simulink model "Ambient_TestBed_org"  (Simulink 10.0)
settings: Solver=FixedStepDiscrete  StartTime=0.0  StopTime=1  FixedStep=1  RelTol=1e-3  EnableMultiTasking=on
undefined symbols (not defined in the file): MWS
libraries: Lib_Turbo_Ambient_TMATS x1
settings Model: Creator=jwchapm2  LastModifiedBy=bhisma
settings DataIOCC: LimitDataPoints=on
settings OptimizationCC: ExpressionDepthLimit=2147483647
settings DebuggingCC: SolverPrmCheckMsg=warning  StateNameClashWarn=warning
settings GRTTargetCC: GeneratePreprocessorConditionals=Disable all  CombineOutputUpdateFcns=on  GRTInterface=off
settings ConfigComp: CovExternalEMLEnable=off

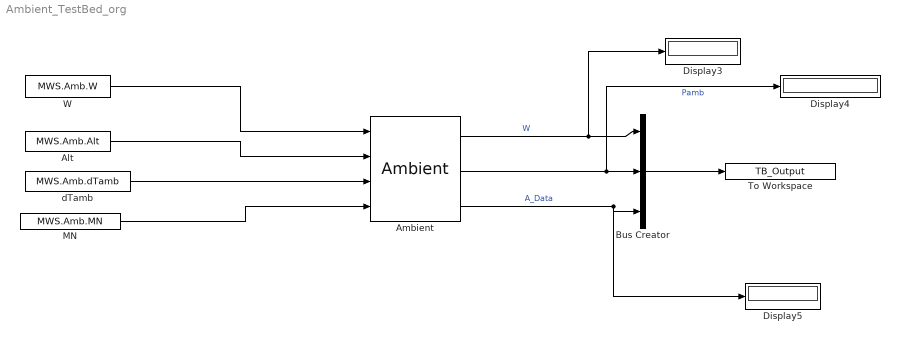
== system Ambient_TestBed_org ==
  Alt : Constant  Value=MWS.Amb.Alt
  Ambient : Lib_Turbo_Ambient_TMATS/Ambient  X_A_AltVec_M=5000*[-1 0 1 2 3 4 5 6 7 8 9 10 12 14 16]  T_A_TsVec_M=[536.51 518.67 500.84 483.03 465.22 447.41 429.62 411.84 394.06 389.97 389.97 389.97 389.97 392.25 397.69]  T_A_PsVec_M=[17.554 14.696 12.228 10.108 8.297 6.759 5.461 4.373 3.468 2.73 2.149 1.692 1.049 0.651 0.406]  AFARc_M=0
  Bus Creator : BusCreator  Inputs=3
  Display3 : Display
  Display4 : Display
  Display5 : Display
  MN : Constant  Value=MWS.Amb.MN
  To Workspace : ToWorkspace  VariableName=TB_Output  SampleTime=-1
  W : Constant  Value=MWS.Amb.W
  dTamb : Constant  Value=MWS.Amb.dTamb
  wires:
  W/1 -> Ambient/1
  dTamb/1 -> Ambient/3
  Ambient/1 -> Bus Creator/1, Display3/1  "W"
  Ambient/2 -> Bus Creator/2, Display4/1  "Pamb"
  Ambient/3 -> Display5/1, Bus Creator/3  "A_Data"
  Bus Creator/1 -> To Workspace/1
  MN/1 -> Ambient/4
  Alt/1 -> Ambient/2
